simulink model "relative_DC_SK"  (R2021a)
settings: Solver=VariableStepAuto  StartTime=0.0  StopTime=time_sim*24  FixedStep=1  RelTol=1e-5
undefined symbols (not defined in the file or in its folder): e, init_conds, n, reference_conds
libraries: pid_lib x2
settings Model: Creator=danie  LastModifiedBy=danie
settings SolverCC: AlgebraicLoopSolver=TrustRegion
settings DebuggingCC: SFMachineParentedDataDiag=warning

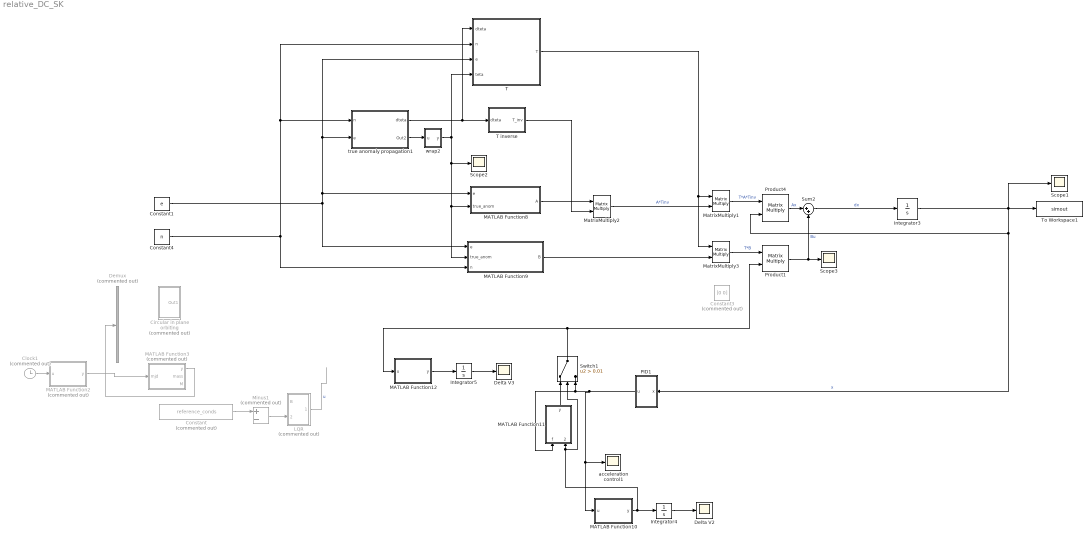
== system relative_DC_SK ==
  Circular in plane orbiting : Subsystem  Commented=on
  Clock1 : Clock  Commented=on
  Constant : Constant  Commented=on  Value=reference_conds
  Constant1 : Constant  Value=e
  Constant3 : Constant  Commented=on  Value=[0 0]
  Constant4 : Constant  Value=n
  Delta V2 : Scope
  Delta V3 : Scope
  Demux : Demux  Commented=on  Outputs=6
  Integrator3 : Integrator  InitialCondition=init_conds
  Integrator4 : Integrator
  Integrator5 : Integrator
  LQR : Subsystem  Commented=on
  MATLAB Function10 : MATLAB Function  TreatAsAtomicUnit=on
  MATLAB Function11 : MATLAB Function  TreatAsAtomicUnit=on
  MATLAB Function12 : MATLAB Function  TreatAsAtomicUnit=on
  MATLAB Function2 : MATLAB Function  Commented=on  TreatAsAtomicUnit=on
  MATLAB Function3 : MATLAB Function  Commented=on  TreatAsAtomicUnit=on
  MATLAB Function8 : MATLAB Function  TreatAsAtomicUnit=on
  MATLAB Function9 : MATLAB Function  TreatAsAtomicUnit=on
  MatrixMultiply1 : Product  Multiplication=Matrix(*)
  MatrixMultiply2 : Product  Multiplication=Matrix(*)
  MatrixMultiply3 : Product  Multiplication=Matrix(*)
  Minus1 : Sum  Commented=on  Inputs=+-
  PID1 : Subsystem
  Product1 : Product  SCDEnableBlockLinearizationSpecification=on  Multiplication=Matrix(*)
  Product4 : Product  SCDEnableBlockLinearizationSpecification=on  Multiplication=Matrix(*)
  Scope1 : Scope
  Scope2 : Scope
  Scope3 : Scope
  Sum2 : Sum  Inputs=|++
  Switch1 : Switch  Criteria=u2 > Threshold  Threshold=0.01
  T : MATLAB Function  TreatAsAtomicUnit=on
  T inverse : MATLAB Function  TreatAsAtomicUnit=on
  To Workspace1 : ToWorkspace  VariableName=simout  SaveFormat=Timeseries  SampleTime=-1
  acceleration control1 : Scope
  true anomaly propagation1 : Subsystem
  wrap2 : MATLAB Function  TreatAsAtomicUnit=on
  wires:
  MATLAB Function2/1(y) -> MATLAB Function3/1(mjd)
  MATLAB Function3/1(y) -> Demux/1
  Clock1/1 -> MATLAB Function2/1(u)
  LQR/1(Out1) -> ?  "u"
  Minus1/1 -> LQR/2(In2)
  Constant/1 -> Minus1/1
  true anomaly propagation1/1(dteta) -> T/1(dteta), T inverse/1(dteta)
  true anomaly propagation1/2(Out2) -> wrap2/1(u)
  MATLAB Function9/1(B) -> MatrixMultiply3/2
  MatrixMultiply1/1 -> Product4/1  "T*A*Tinv"
  Sum2/1 -> Integrator3/1  "dx"
  T inverse/1(T_inv) -> MatrixMultiply2/2
  Product1/1 -> Sum2/2, Scope3/1  "Bu"
  Product4/1 -> Sum2/1  "Ax"
  Constant1/1 -> MATLAB Function9/1(e), T/3(e), true anomaly propagation1/2(e), MATLAB Function8/1(e)
  Constant4/1 -> MATLAB Function9/3(n), T/2(n), true anomaly propagation1/1(n)
  MATLAB Function8/1(A) -> MatrixMultiply2/1
  MatrixMultiply3/1 -> Product1/1  "T*B"
  T/1(T) -> MatrixMultiply3/1, MatrixMultiply1/1
  wrap2/1(y) -> Scope2/1, MATLAB Function9/2(true_anom), MATLAB Function8/2(true_anom), T/4(teta)
  MatrixMultiply2/1 -> MatrixMultiply1/2  "A*Tinv"
  MATLAB Function12/1(y) -> Integrator5/1
  Integrator5/1 -> Delta V3/1
  PID1/1(u) -> MATLAB Function11/1(f), Switch1/3, MATLAB Function10/1(u), acceleration control1/1
  MATLAB Function11/1(y) -> Switch1/1
  Integrator3/1 -> Scope1/1, To Workspace1/1, PID1/1(x), Product4/2  "x"
  MATLAB Function10/1(y) -> MATLAB Function11/2(norm_f), Switch1/2, Integrator4/1
  Integrator4/1 -> Delta V2/1
  Switch1/1 -> MATLAB Function12/1(u), Product1/2

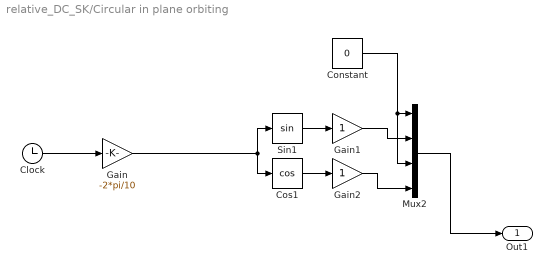
== system relative_DC_SK/Circular in plane orbiting ==
  Clock : Clock
  Constant : Constant  Value=0
  Cos1 : Trigonometry  Operator=cos
  Gain : Gain  Gain=-2*pi/10
  Gain1 : Gain
  Gain2 : Gain
  Mux2 : Mux
  Sin1 : Trigonometry
  Out1 : Outport
  wires:
  Gain/1 -> Cos1/1, Sin1/1
  Gain2/1 -> Mux2/4
  Clock/1 -> Gain/1
  Sin1/1 -> Gain1/1
  Cos1/1 -> Gain2/1
  Mux2/1 -> Out1/1
  Gain1/1 -> Mux2/2
  Constant/1 -> Mux2/3, Mux2/1

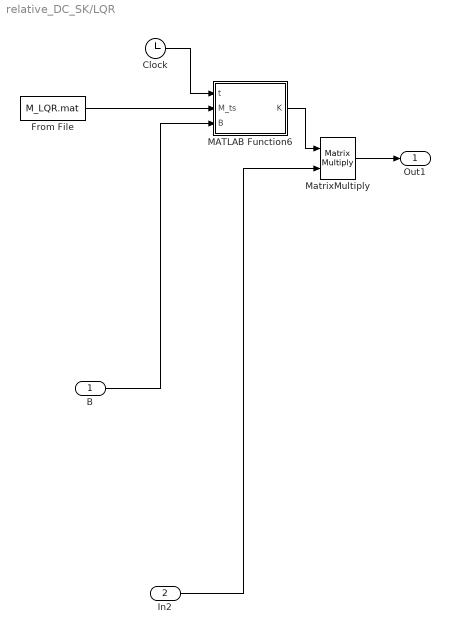
== system relative_DC_SK/LQR ==
  B : Inport
  In2 : Inport  Port=2
  Clock : Clock
  From File : FromFile  FileName=M_LQR.mat  SampleTime=0
  MATLAB Function6 : MATLAB Function  TreatAsAtomicUnit=on
  MatrixMultiply : Product  Multiplication=Matrix(*)
  Out1 : Outport
  wires:
  MATLAB Function6/1(K) -> MatrixMultiply/1
  From File/1 -> MATLAB Function6/2(M_ts)
  Clock/1 -> MATLAB Function6/1(t)
  MatrixMultiply/1 -> Out1/1
  B/1 -> MATLAB Function6/3(B)
  In2/1 -> MatrixMultiply/2

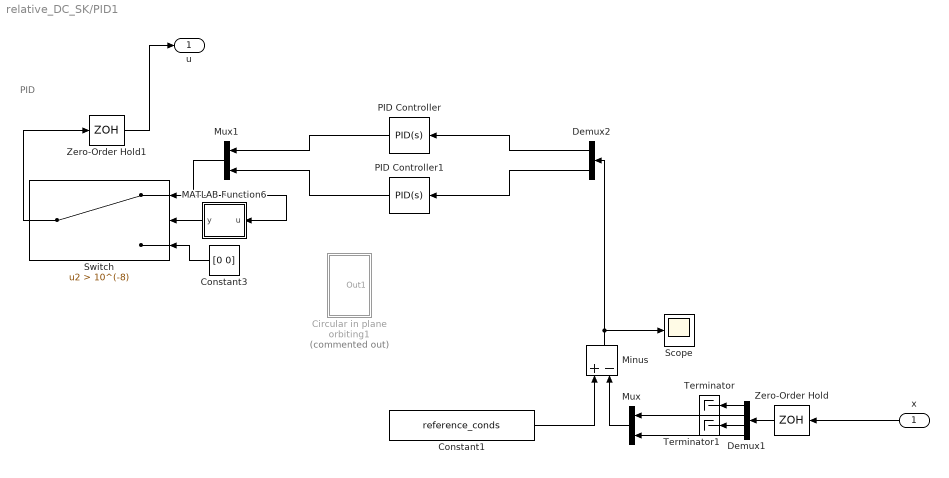
== system relative_DC_SK/PID1 ==
  note: PID
  x : Inport
  Circular in plane orbiting1 : Subsystem  Commented=on
  Constant1 : Constant  Value=reference_conds
  Constant3 : Constant  Value=[0 0]
  Demux1 : Demux
  Demux2 : Demux  Outputs=2
  MATLAB Function6 : MATLAB Function  TreatAsAtomicUnit=on
  Minus : Sum  Inputs=+-
  Mux : Mux  Inputs=2
  Mux1 : Mux  Inputs=2
  PID Controller : pid_lib/PID Controller  Controller=PID  Form=Parallel  TimeDomain=Continuous-time  UseExternalTs=off  SampleTime=-1  IntegratorMethod=Forward Euler  FilterMethod=Forward Euler  ControllerParametersSource=internal  P=0.462311792556731  I=0.00231107700783669  D=20.4098555311429  UseFilter=on  N=0.839478741530513  TunerSelectOption=Transfer Function Based (PID Tuner App)  InitialConditionSource=internal  InitialConditionForIntegrator=0  InitialConditionForFilter=0  DifferentiatorICPrevScaledInput=0  ExternalReset=none  TrackingMode=off  Kt=1  LimitOutput=off  SatLimitsSource=internal  UpperSaturationLimit=inf  LowerSaturationLimit=-inf  LinearizeAsGain=on  AntiWindupMode=none  Kb=1  POutMin=[]  POutMax=[]  IOutMin=[]  IOutMax=[]  DOutMin=[]  DOutMax=[]  NOutMin=[]  NOutMax=[]  SumOutMin=[]  SumOutMax=[]  SaturationOutMin=[]  SaturationOutMax=[]  PParamMin=[]  PParamMax=[]  IParamMin=[]  IParamMax=[]  DParamMin=[]  DParamMax=[]  NParamMin=[]  NParamMax=[]  KbParamMin=[]  KbParamMax=[]  KtParamMin=[]  KtParamMax=[]  KbOutMin=[]  KbOutMax=[]  KtOutMin=[]  KtOutMax=[]  IntegratorOutMin=[]  IntegratorOutMax=[]  FilterOutMin=[]  FilterOutMax=[]  SumI1OutMin=[]  SumI1OutMax=[]  SumI2OutMin=[]  SumI2OutMax=[]  SumI3OutMin=[]  SumI3OutMax=[]  SumI4OutMin=[]  SumI4OutMax=[]  SumDOutMin=[]  SumDOutMax=[]  DifferentiatorOutMin=[]  DifferentiatorOutMax=[]  FilterDiffOutCoefMin=[]  FilterDiffOutCoefMax=[]  ReciprocalOutMin=[]  ReciprocalOutMax=[]  SumDenOutMin=[]  SumDenOutMax=[]  SumNumOutMin=[]  SumNumOutMax=[]  DivideOutMin=[]  DivideOutMax=[]  UdiffTsProdOutMin=[]  UdiffTsProdOutMax=[]  NTsProdOutMin=[]  NTsProdOutMax=[]  UintegralTsProdOutMin=[]  UintegralTsProdOutMax=[]  UngainTsProdOutMin=[]  UngainTsProdOutMax=[]  IntegratorContinuousStateAttributes=''  IntegratorStateMustResolveToSignalObject=off  IntegratorRTWStateStorageClass=Auto  FilterContinuousStateAttributes=''  FilterStateMustResolveToSignalObject=off  FilterRTWStateStorageClass=Auto  ParallelPVariant=InternalParameters  IdealPVariant=Disabled  IVariant=InternalParameters  DVariant=InternalParameters  IntegratorVariant=Continuous  SatVariant=Disabled  AWVariant=Passthrough  PCopyVariant=Disabled  TRVariant=Disabled  FdbkBlocksVariant=Forward  IdealPFdbkVariant=Disabled  SatFdbkVariant=Disabled  DerivativeFilterVariant=ContFilter  NVariant=InternalParameters  NCopyVariant=Disabled  FilterICVariant=InternalICsFilter  IntegratorICVariant=InternalICs  ExternalResetVariant=Disabled  TRSumVariant=Passthrough  SumFdbkVariant=Disabled  SumVariant=Sum_PID  TsampFilterVariant=InternalTs  TsampNgainVariant=Passthrough  TsampIntegralVariant=Passthrough  ExternalSaturationOutDataTypeStr=Inherit: Same as second input
  PID Controller1 : pid_lib/PID Controller  Controller=PID  Form=Parallel  TimeDomain=Continuous-time  UseExternalTs=off  SampleTime=-1  IntegratorMethod=Forward Euler  FilterMethod=Forward Euler  ControllerParametersSource=internal  P=2.47188926696688  I=0.00241892232645916  D=572.134688671861  UseFilter=on  N=0.0355273565337747  TunerSelectOption=Transfer Function Based (PID Tuner App)  InitialConditionSource=internal  InitialConditionForIntegrator=0  InitialConditionForFilter=0  DifferentiatorICPrevScaledInput=0  ExternalReset=none  TrackingMode=off  Kt=1  LimitOutput=off  SatLimitsSource=internal  UpperSaturationLimit=inf  LowerSaturationLimit=-inf  LinearizeAsGain=on  AntiWindupMode=none  Kb=1  POutMin=[]  POutMax=[]  IOutMin=[]  IOutMax=[]  DOutMin=[]  DOutMax=[]  NOutMin=[]  NOutMax=[]  SumOutMin=[]  SumOutMax=[]  SaturationOutMin=[]  SaturationOutMax=[]  PParamMin=[]  PParamMax=[]  IParamMin=[]  IParamMax=[]  DParamMin=[]  DParamMax=[]  NParamMin=[]  NParamMax=[]  KbParamMin=[]  KbParamMax=[]  KtParamMin=[]  KtParamMax=[]  KbOutMin=[]  KbOutMax=[]  KtOutMin=[]  KtOutMax=[]  IntegratorOutMin=[]  IntegratorOutMax=[]  FilterOutMin=[]  FilterOutMax=[]  SumI1OutMin=[]  SumI1OutMax=[]  SumI2OutMin=[]  SumI2OutMax=[]  SumI3OutMin=[]  SumI3OutMax=[]  SumI4OutMin=[]  SumI4OutMax=[]  SumDOutMin=[]  SumDOutMax=[]  DifferentiatorOutMin=[]  DifferentiatorOutMax=[]  FilterDiffOutCoefMin=[]  FilterDiffOutCoefMax=[]  ReciprocalOutMin=[]  ReciprocalOutMax=[]  SumDenOutMin=[]  SumDenOutMax=[]  SumNumOutMin=[]  SumNumOutMax=[]  DivideOutMin=[]  DivideOutMax=[]  UdiffTsProdOutMin=[]  UdiffTsProdOutMax=[]  NTsProdOutMin=[]  NTsProdOutMax=[]  UintegralTsProdOutMin=[]  UintegralTsProdOutMax=[]  UngainTsProdOutMin=[]  UngainTsProdOutMax=[]  IntegratorContinuousStateAttributes=''  IntegratorStateMustResolveToSignalObject=off  IntegratorRTWStateStorageClass=Auto  FilterContinuousStateAttributes=''  FilterStateMustResolveToSignalObject=off  FilterRTWStateStorageClass=Auto  ParallelPVariant=InternalParameters  IdealPVariant=Disabled  IVariant=InternalParameters  DVariant=InternalParameters  IntegratorVariant=Continuous  SatVariant=Disabled  AWVariant=Passthrough  PCopyVariant=Disabled  TRVariant=Disabled  FdbkBlocksVariant=Forward  IdealPFdbkVariant=Disabled  SatFdbkVariant=Disabled  DerivativeFilterVariant=ContFilter  NVariant=InternalParameters  NCopyVariant=Disabled  FilterICVariant=InternalICsFilter  IntegratorICVariant=InternalICs  ExternalResetVariant=Disabled  TRSumVariant=Passthrough  SumFdbkVariant=Disabled  SumVariant=Sum_PID  TsampFilterVariant=InternalTs  TsampNgainVariant=Passthrough  TsampIntegralVariant=Passthrough  ExternalSaturationOutDataTypeStr=Inherit: Same as second input
  Scope : Scope
  Switch : Switch  Criteria=u2 > Threshold  Threshold=10^(-8)
  Terminator : Terminator
  Terminator1 : Terminator
  Zero-Order Hold : ZeroOrderHold
  Zero-Order Hold1 : ZeroOrderHold
  u : Outport
  wires:
  Minus/1 -> Demux2/1, Scope/1
  Zero-Order Hold/1 -> Demux1/1
  Demux1/2 -> Mux/1
  Demux2/2 -> PID Controller1/1
  PID Controller1/1 -> Mux1/2
  Mux/1 -> Minus/2
  MATLAB Function6/1(y) -> Switch/2
  Mux1/1 -> Switch/1, MATLAB Function6/1(u)
  Demux1/4 -> Mux/2
  Constant3/1 -> Switch/3
  Switch/1 -> Zero-Order Hold1/1
  Demux2/1 -> PID Controller/1
  PID Controller/1 -> Mux1/1
  x/1 -> Zero-Order Hold/1
  Zero-Order Hold1/1 -> u/1
  Demux1/1 -> Terminator/1
  Demux1/3 -> Terminator1/1
  Constant1/1 -> Minus/1

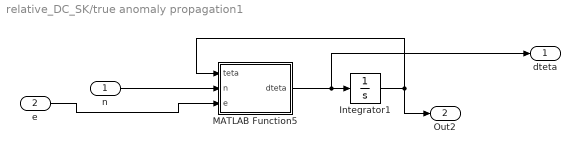
== system relative_DC_SK/true anomaly propagation1 ==
  n : Inport
  e : Inport  Port=2
  Integrator1 : Integrator
  MATLAB Function5 : MATLAB Function  TreatAsAtomicUnit=on
  dteta : Outport
  Out2 : Outport  Port=2
  wires:
  MATLAB Function5/1(dteta) -> dteta/1, Integrator1/1
  e/1 -> MATLAB Function5/3(e)
  Integrator1/1 -> Out2/1, MATLAB Function5/1(teta)
  n/1 -> MATLAB Function5/2(n)

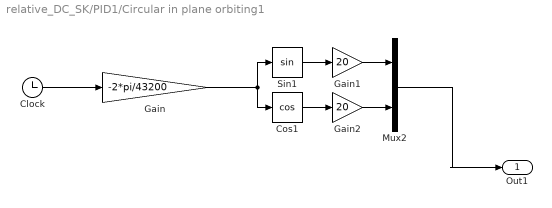
== system relative_DC_SK/PID1/Circular in plane orbiting1 ==
  Clock : Clock
  Cos1 : Trigonometry  Operator=cos
  Gain : Gain  Gain=-2*pi/43200
  Gain1 : Gain  Gain=20
  Gain2 : Gain  Gain=20
  Mux2 : Mux  Inputs=2
  Sin1 : Trigonometry
  Out1 : Outport
  wires:
  Gain/1 -> Cos1/1, Sin1/1
  Gain2/1 -> Mux2/2
  Clock/1 -> Gain/1
  Sin1/1 -> Gain1/1
  Cos1/1 -> Gain2/1
  Gain1/1 -> Mux2/1
  Mux2/1 -> Out1/1

== matlab function relative_DC_SK/MATLAB Function12 ==
  data: u input; y output
function y = fcn(u)

y =norm(u);

== matlab function relative_DC_SK/PID1/MATLAB Function6 ==
  data: u input; y output
function y = fcn(u)

y = norm(u);

== matlab function relative_DC_SK/MATLAB Function2 ==
  data: u input; y output
function y = time_conv(u)
y=double(60676+((u/3600)/24));

== matlab function relative_DC_SK/MATLAB Function3 ==
  data: mjd input; y output; mass output; M output
function [y, mass, M]= get_eph(mjd)
    [y, mass, M]=ephNEO(mjd,28);

== matlab function relative_DC_SK/LQR/MATLAB Function6 ==
  data: t input; M_ts input; K output; B input
function K = fcn(t,M_ts,B)
flag=0;
% for i=1:(length(M_ts.Time)-1)
%     if and(t>=M_ts.Time(i),t<M_ts.Time(i+1))
%         M=M_ts.data(i);
%         flag=1;
%         break
%     else
%         M=zeros(4,4)
%     end
% end
M=reshape(M_ts,4,4);
K=-B.'*M;

== matlab function relative_DC_SK/MATLAB Function8 ==
  data: e input; A output; true_anom input
function A = A_ss(e,true_anom)
A=[ 2*e*sin(true_anom)/(1+e*cos(true_anom)), (3+e*cos(true_anom))/(1+e*cos(true_anom)), 2, -2*e*sin(true_anom)/(1+e*cos(true_anom)); 
    1, 0, 0, 0;
   -2, 2*e*sin(true_anom)/(1+e*cos(true_anom)), 2*e*sin(true_anom)/(1+e*cos(true_anom)), e*cos(true_anom)/(1+e*cos(true_anom));
   0, 0, 1, 0];

== matlab function relative_DC_SK/MATLAB Function9 ==
  data: e input; B output; true_anom input; n input
function B = B_ss(e,true_anom,n)
B=((1-(e^2))^3)/(((1+e*cos(true_anom))^4)*(n^2))*[1 0; 0 0; 0 1; 0 0];

== matlab function relative_DC_SK/T ==
  data: dteta input; T output; n input; e input; teta input
function T = fcn(dteta, n,e,teta)
T=[dteta^2 dteta*(-(n*2*(1+e*cos(teta))*e*sin(teta)/((1-e^2)^1.5))) 0 0; 0 dteta 0 0; 0 0 dteta^2 dteta*(-(n*2*(1+e*cos(teta))*e*sin(teta)/((1-e^2)^1.5))); 0 0 0 dteta];

== matlab function relative_DC_SK/T inverse ==
  data: dteta input; T_inv output
function T_inv = fcn(dteta)
T_inv=[1/dteta 0 0 0; 0 1 0 0; 0 0 1/dteta 0; 0 0 0 1];

== matlab function relative_DC_SK/true anomaly propagation1/MATLAB Function5 ==
  data: teta input; n input; dteta output; e input
function dteta = fcn(teta,n,e)
dteta=(n*(1+e*cos(teta))^2)/((1-e^2)^1.5);

== matlab function relative_DC_SK/wrap2 ==
  data: u input; y output
function y = fcn(u)

y = mod(u,2*pi);

== matlab function relative_DC_SK/MATLAB Function10 ==
  data: u input; y output
function y = fcn(u)

y =norm(u);

== matlab function relative_DC_SK/MATLAB Function11 ==
  data: f input; y output; norm_f input
function y = fcn(f,norm_f)
y=[f(1)/norm_f; f(2)/norm_f].*0.01;
